simulink subsystem "Pure_Pursuit_Lat"  (R2022b)
settings: Solver=VariableStepAuto  StartTime=0.0  StopTime=10.0  RelTol=1e-3
undefined symbols (not defined in the file): route1_waypoint_raw
libraries: CarMaker4SL x8
settings Model: Creator=User  LastModifiedBy=USER

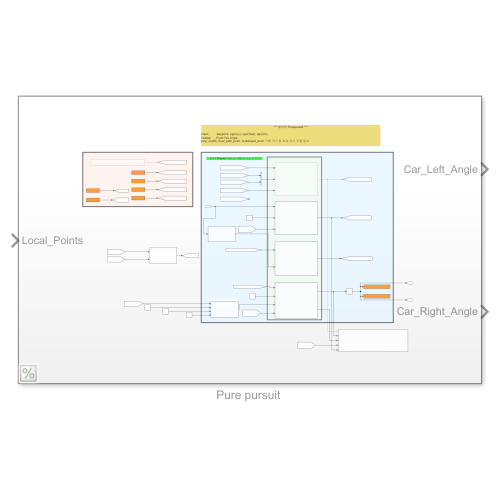
[thumbnail: Simulink's stored preview of the top-level diagram]
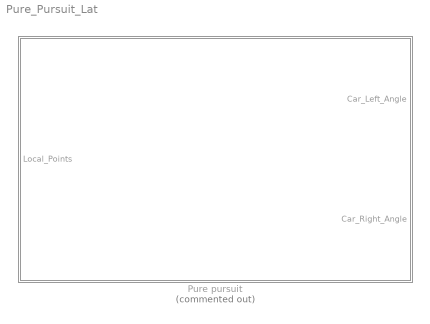
== system Pure_Pursuit_Lat ==
  "Pure pursuit " : Subsystem  Commented=on

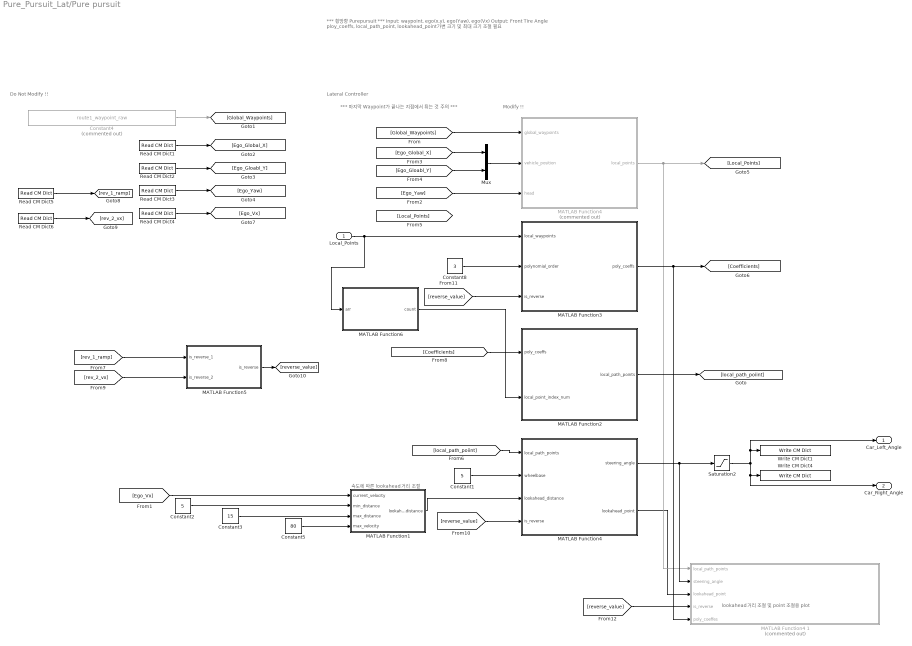
== system Pure_Pursuit_Lat/Pure pursuit  ==
  note: Do Not Modify !!
  note: 속도에 따른 lookahead 거리 조절
  note: Modify !!
  note: Lateral Controller
  note: *** 마지막 Waypoint가 끝나는 지점에서 튀는 것 주의 ***
  note: lookahead 거리 조절 및 point 조절용 plot
  note: *** 횡방향 Purepursuit ***
      |
      | Input: waypoint, ego(x,y), ego(Yaw), ego(Vx)
      | Output: Front Tire Angle
      | ploy_coeffs, local_path_point, lookahead_point 가변 크기 및 최대 크기 조절 필요
  Local_Points : Inport
  Constant1 : Constant  Value=5
  Constant2 : Constant  Value=5
  Constant3 : Constant  Value=15
  Constant4 : Constant  Commented=on  Value=route1_waypoint_raw
  Constant5 : Constant  Value=80
  Constant8 : Constant  Value=3
  MATLAB Function1 : MATLAB Function  TreatAsAtomicUnit=on
  MATLAB Function2 : MATLAB Function  TreatAsAtomicUnit=on
  MATLAB Function3 : MATLAB Function  TreatAsAtomicUnit=on
  MATLAB Function4 : MATLAB Function  TreatAsAtomicUnit=on
  "MATLAB Function4 " : MATLAB Function  Commented=on  TreatAsAtomicUnit=on
  MATLAB Function4 1 : MATLAB Function  Commented=on  TreatAsAtomicUnit=on
  MATLAB Function5 : MATLAB Function  TreatAsAtomicUnit=on
  MATLAB Function6 : MATLAB Function  TreatAsAtomicUnit=on
  Mux : Mux  Inputs=2
  Read CM Dict1 : CarMaker4SL/Read CM Dict  xname=Car.Fr1.tx  xsync=off  xstime=Inherited
  Read CM Dict2 : CarMaker4SL/Read CM Dict  xname=Car.Fr1.ty  xsync=off  xstime=Inherited
  Read CM Dict3 : CarMaker4SL/Read CM Dict  xname=Car.Fr1.rz  xsync=off  xstime=Inherited
  Read CM Dict4 : CarMaker4SL/Read CM Dict  xname=Car.v  xsync=off  xstime=Inherited
  Read CM Dict5 : CarMaker4SL/Read CM Dict  xname=VC.Lights.Reverse  xsync=off  xstime=Inherited
  Read CM Dict6 : CarMaker4SL/Read CM Dict  xname=Car.vx  xsync=off  xstime=Inherited
  Saturation2 : Saturate  UpperLimit=10  LowerLimit=-10
  Write CM Dict1 : CarMaker4SL/Write CM Dict  xname=Car.CFL.rz_ext  xsync=off
  Write CM Dict4 : CarMaker4SL/Write CM Dict  xname=Car.CFR.rz_ext  xsync=off
  Car_Left_Angle : Outport
  Car_Right_Angle : Outport  Port=2
  wires:
  [reverse_value] -> MATLAB Function4 1/4(is_reverse)
  MATLAB Function1/1(lookahead_distance) -> MATLAB Function4/3(lookahead_distance)
  MATLAB Function4/2(lookahead_point) -> MATLAB Function4 1/3(lookahead_point)
  [rev_2_vx] -> MATLAB Function5/2(is_reverse_2)
  "MATLAB Function4 "/1(local_points) -> [Local_Points], MATLAB Function4 1/1(local_path_points)
  [reverse_value] -> MATLAB Function4/4(is_reverse)
  Mux/1 -> "MATLAB Function4 "/2(vehicle_position)
  Read CM Dict2/1 -> [Ego_Gloabl_Y]
  Read CM Dict6/1 -> [rev_2_vx]
  Constant3/1 -> MATLAB Function1/3(max_distance)
  Constant5/1 -> MATLAB Function1/4(max_velocity)
  MATLAB Function5/1(is_reverse) -> [reverse_value]
  MATLAB Function4/1(steering_angle) -> MATLAB Function4 1/2(steering_angle), Saturation2/1
  Constant2/1 -> MATLAB Function1/2(min_distance)
  [Ego_Gloabl_Y] -> Mux/2
  Read CM Dict5/1 -> [rev_1_ramp]
  Read CM Dict1/1 -> [Ego_Global_X]
  [Coefficients] -> MATLAB Function2/1(poly_coeffs)
  [Ego_Global_X] -> Mux/1
  Read CM Dict4/1 -> [Ego_Vx]
  [Global_Waypoints] -> "MATLAB Function4 "/1(global_waypoints)
  Constant8/1 -> MATLAB Function3/2(polynomial_order)
  Constant1/1 -> MATLAB Function4/2(wheelbase)
  [local_path_poiint] -> MATLAB Function4/1(local_path_points)
  [rev_1_ramp] -> MATLAB Function5/1(is_reverse_1)
  MATLAB Function3/1(poly_coeffs) -> [Coefficients], MATLAB Function4 1/5(poly_coeffes)
  [Ego_Vx] -> MATLAB Function1/1(current_velocity)
  [reverse_value] -> MATLAB Function3/3(is_reverse)
  MATLAB Function2/1(local_path_points) -> [local_path_poiint]
  Read CM Dict3/1 -> [Ego_Yaw]
  [Ego_Yaw] -> "MATLAB Function4 "/3(head)
  Saturation2/1 -> Car_Left_Angle/1, Write CM Dict1/1, Car_Right_Angle/1, Write CM Dict4/1
  Local_Points/1 -> MATLAB Function6/1(arr), MATLAB Function3/1(local_waypoints)
  MATLAB Function6/1(count) -> MATLAB Function2/2(local_point_index_num)
  Constant4/1 -> [Global_Waypoints]

== matlab function Pure_Pursuit_Lat/Pure pursuit /MATLAB Function1 ==
  settings: updateMethod=DISCRETE  sampleTime=0.05
  data: current_velocity input; min_distance input; lookahead_distance output; max_distance input; max_velocity input
function lookahead_distance = calculate_lookahead_distance(current_velocity, min_distance, max_distance, max_velocity)
    % current_velocity: 현재 차량의 속도 [m/s]
    % min_distance: 최소 lookahead 거리 [m]
    % max_distance: 최대 lookahead 거리 [m]
    % max_velocity: 최대 속도 [m/s], 해당 속도에서 max_distance를 사용

    % lookahead 거리를 속도에 비례하여 계산
    lookahead_distance = min_distance + (max_distance - min_distance) * (current_velocity / max_velocity);

    % lookahead 거리가 최소와 최대 사이의 값으로 유지되도록 제한
    lookahead_distance = max(min_distance, min(lookahead_distance, max_distance));
end

== matlab function Pure_Pursuit_Lat/Pure pursuit /MATLAB Function2 ==
  settings: updateMethod=DISCRETE  sampleTime=0.05
  data: poly_coeffs input; local_path_points output size=[100000,2]; local_point_index_num input
function local_path_points = calculate_polynomial_values(poly_coeffs,local_point_index_num)
    % 다항식 계수들이 poly_coeffs로 입력되었는지 확인합니다.
    if isempty(poly_coeffs)
        error('poly_coeffs is empty. Make sure to pass the polynomial coefficients.');
    end

    % x_values를 로컬 좌표계에서 사용할 범위로 설정
    x_values = -2:0.1:local_point_index_num-2;
    
    % 다항식 계수를 사용해 y 값을 계산
    y_values = polyval(poly_coeffs(1, :), x_values);
    
    % x와 y 값을 결합하여 [x, y] 형식의 로컬 경로 포인트 생성
    local_path_points = [x_values', y_values'];
    
    % 로컬 경로 포인트의 크기 고정 (예: 최대 크기 [1000, 2])
    max_size = 100;
    if size(local_path_points, 1) > max_size
        local_path_points = local_path_points(1:max_size, :);
    end
end

== matlab function Pure_Pursuit_Lat/Pure pursuit /MATLAB Function3 ==
  settings: updateMethod=DISCRETE  sampleTime=0.05
  data: local_waypoints input; poly_coeffs output size=[10000,7]; polynomial_order input; is_reverse input
function poly_coeffs = fit_polynomial_segments(local_waypoints, polynomial_order,is_reverse)


%indxs = findClosetWayPoints(local_waypoints(:,1),local_waypoints(:,2),10,is_reverse);

indxs = findClosetWayPoints(local_waypoints(:,1),local_waypoints(:,2),10);
%disp(indxs)
if is_reverse == true   
    poly_coeffs = polyfit(local_waypoints(indxs-5,1), local_waypoints(indxs-5,2), polynomial_order);
else 
    poly_coeffs = polyfit(local_waypoints(indxs,1), local_waypoints(indxs,2), polynomial_order);
end
%disp(poly_coeffs)
%             poly_coeffs = polyfit(local_waypoints(indxs,1), local_waypoints(indxs,2), polynomial_order);
          

end


function [ids] = findClosetWayPoints(x, y, np) %is_reverse)
    dummy = (x.^2 + y.^2);
    [~, id] = min(dummy);
    max_id = length(x);

%     if (is_reverse==true)
%         % 역방향일 때: 뒤쪽 웨이포인트들을 선택 (id부터 id-np+1까지)
%         ids = max(1, id-np+1):id; % 최소값이 1보다 작아지지 않도록 보정
%         %ids = flip(ids);
%     else
%         % 전진일 때: 앞쪽 웨이포인트들을 선택 (id부터 id+np-1까지)
%         ids = id:min(id+np-1, max_id);
%         
%     end

    ids = id:min(id+np-1, max_id);

end

== matlab function Pure_Pursuit_Lat/Pure pursuit /MATLAB Function4 ==
  settings: updateMethod=DISCRETE  sampleTime=0.05
  data: local_path_points input; steering_angle output; wheelbase input; lookahead_distance input; lookahead_point output size=[1,2]; is_reverse input
function [steering_angle, lookahead_point] = pure_pursuit_controller(local_path_points, wheelbase, lookahead_distance, is_reverse)
% 초기화: lookahead_point의 크기를 명시적으로 지정
lookahead_point = NaN(1, 2);

if (is_reverse == true)
    lookahead_distance = lookahead_distance / 1.5; % 후진 시 거리를 줄여서 사용
    for i = 20:-1:1
        disp("backward")
        disp(i)
        distance = norm(local_path_points(i, :) - [0, 0]);
        disp(distance)
        if distance >= lookahead_distance
            lookahead_point = local_path_points(i, :);
            break;
        end
    end

else
    % 전진 시, 차량의 앞쪽 포인트들을 탐색
    for i = 1:size(local_path_points, 1)
        disp("forward")
        disp(i)

        distance = norm(local_path_points(i, :));
        disp(distance)
        if distance >= lookahead_distance
            lookahead_point = local_path_points(i, :);
            break;
        end
    end
end

% 만약 lookahead 거리를 만족하는 포인트가 없다면, 마지막 포인트를 사용
if any(isnan(lookahead_point))
    if (is_reverse == true)
        lookahead_point = local_path_points(1, :); % 후진 시 가장 첫 번째 포인트
        disp("Selected first point for reverse:")
        disp(lookahead_point)
    else
        lookahead_point = local_path_points(end, :); % 전진 시 먼 포인트
        disp("Selected farthest point for forward:")
        disp(lookahead_point)
    end
end

% 조향각 계산 (후진 시 부호 반전 고려)
% alpha = atan2(lookahead_point(2), lookahead_point(1)); % lookahead point 기준 각도
if (is_reverse == true)
    alpha = atan2(-lookahead_point(2), -lookahead_point(1)); % lookahead point 기준 각도
else
    alpha = atan2(lookahead_point(2), lookahead_point(1)); % lookahead point 기준 각도
end
Ld = norm(lookahead_point); % lookahead point와의 거리

% 후진 시 조향각을 반대로 계산
if (is_reverse == true)
    steering_angle = -atan2(2 * wheelbase * sin(alpha), Ld);
else
    steering_angle = atan2(2 * wheelbase * sin(alpha), Ld);
end
end

== matlab function Pure_Pursuit_Lat/Pure pursuit /MATLAB Function4  ==
  settings: updateMethod=DISCRETE  sampleTime=0.05
  data: global_waypoints input; local_points output; vehicle_position input; head input
function local_points = global_to_local_waypoints(global_waypoints, vehicle_position, head)
    % global_waypoints: Nx2 행렬로, 각 행은 [x, y] 형식의 글로벌 웨이포인트 좌표
    % vehicle_position: [x, y] 형식의 차량의 현재 글로벌 좌표
    % head: 차량의 헤딩 (Yaw) 값 [rad]
    
    x_vehicle = vehicle_position(1);
    y_vehicle = vehicle_position(2);

    % 회전 행렬 생성 (글로벌에서 로컬로)
    R = [cos(head), sin(head); -sin(head), cos(head)];

    % 각 글로벌 웨이포인트에서 차량 위치를 빼고, 회전 행렬을 적용하여 로컬 좌표로 변환
    local_points = (global_waypoints - [x_vehicle, y_vehicle]) * R';
    
    end

== matlab function Pure_Pursuit_Lat/Pure pursuit /MATLAB Function4 1 ==
  settings: updateMethod=DISCRETE  sampleTime=0.05
  data: local_path_points input; steering_angle input; lookahead_point input; is_reverse input; poly_coeffes input
function plot_local_path_with_lookahead(local_path_points, steering_angle, lookahead_point, is_reverse, poly_coeffes)
    % local_path_points: Nx2 행렬, 로컬 좌표계에서의 경로 포인트
    % steering_angle: 차량의 현재 조향 각도 [rad]
    % lookahead_point: 조향각 계산에 사용된 로컬 좌표계의 lookahead 포인트 [x, y]

    % count 변수를 함수 외부에서 정의하거나, 함수 내부에서 지속적으로 사용할 수 있도록 설정합니다.
    persistent count;
    if isempty(count)
        count = 0;
    end

    % count 값을 증가시킵니다.
    count = count + 1;

    % 3번마다 플롯을 업데이트합니다.
    if mod(count, 3) == 1
        figure(1);
        clf; % 기존 플롯 초기화
        hold on;
        grid on;
        
        
        % x 범위 설정 (x의 값을 원하는 범위로 설정)
        x_values = linspace(-10, 10, 100); % -10에서 10까지 100개의 값을 생성
        
        % 다항식의 y 값 계산
        y_values = polyval(poly_coeffes, x_values);
        
        % 플롯 그리기
        
        
        % 로컬 경로 포인트를 플롯
        plot(local_path_points(:, 1), local_path_points(:, 2), 'b.-', 'DisplayName', 'Local Path Points');

        % 현재 차량 위치 및 조향 각도 표시
        plot(0, 0, 'ro', 'DisplayName', 'Vehicle Position'); % 차량의 위치는 로컬 좌표계에서 (0,0)

        % 조향 각도를 화살표로 표시 (길이를 조정해 가시성을 확보)
        arrow_length = 2.0; % 화살표의 길이 (단위를 맞추어 조정)
        quiver(0, 0, arrow_length * cos(steering_angle), arrow_length * sin(steering_angle), 0, ...
               'r', 'LineWidth', 2, 'MaxHeadSize', 1, 'DisplayName', 'Steering Direction');
        plot(x_values, y_values, 'r-', 'LineWidth', 2,'DisplayName', 'coeff');
        % lookahead 포인트를 플롯 (초록색 별표)
        if (is_reverse == true)
            plot(lookahead_point(1), lookahead_point(2), 'r*', 'MarkerSize', 20, 'DisplayName', 'Lookahead Point');
        else
            plot(lookahead_point(1), lookahead_point(2), 'g*', 'MarkerSize', 10, 'DisplayName', 'Lookahead Point');
            

        % 플롯 설정
        xlabel('X (local frame)');
        ylabel('Y (local frame)');
        axis equal;
        xlim([-50 50]);
        ylim([-50 50]);
        legend('show');

        drawnow; % 실시간 플롯 업데이트
    end
end

== matlab function Pure_Pursuit_Lat/Pure pursuit /MATLAB Function5 ==
  settings: updateMethod=DISCRETE  sampleTime=0.05
  data: is_reverse_1 input; is_reverse_2 input; is_reverse output
function is_reverse = judge_reverse(is_reverse_1,is_reverse_2)
    if is_reverse_1 == 1 && is_reverse_2 < 1
        is_reverse = true;
    else
        is_reverse = false;
    end
end

== matlab function Pure_Pursuit_Lat/Pure pursuit /MATLAB Function6 ==
  settings: updateMethod=DISCRETE  sampleTime=0.05
  data: arr input; count output
function count = getIndexCount(arr)
    % 배열의 길이를 반환하는 함수
    count = length(arr);
end
